simulink model "BMS_V4"  (R2017b)
settings: Solver=FixedStepDiscrete  StartTime=0.0  StopTime=inf  FixedStep=BASETIME  RelTol=1e-3  EnableMultiTasking=on
values from neighbouring files (symbols this model uses):
  AKT_BALANCE = uint16(8)    [BMS_V4_config.m]
  BALANCE = uint16(4)    [BMS_V4_config.m]
  BALANCE_RESISTOR = int32(5)    [BMS_V4_config.m]
  BALANCE_VEC = uint16(8)    [BMS_V4_config.m]
  CELL_SOC = uint16(7)    [BMS_V4_config.m]
  CELL_STATE = uint16(3)    [BMS_V4_config.m]
  CELL_TEMPERATURE = uint16(6)    [BMS_V4_config.m]
  CELL_VOLTAGE = uint16(5)    [BMS_V4_config.m]
  CELLACTBITFIELD = hex2dec('300')    [BMS_V4_config.m]
  CELLDEACTBITFIELD = hex2dec('100')    [BMS_V4_config.m]
  CELLT_BURST = uint16(6)    [BMS_V4_config.m]
  CELLV_BURST = uint16(5)    [BMS_V4_config.m]
  CLK_CYC_timer_1 = 586    [BMS_V4_config.m]
  CLK_CYC_timer_2 = 5860    [BMS_V4_config.m]
  CLK_CYC_timer_3 = 280    [BMS_V4_config.m]
  CLK_CYC_timer_4 = 586*100    (= 58600)    [BMS_V4_config.m]
  CLK_CYC_timer_5 = 5800*2    (= 11600)    [BMS_V4_config.m]
  CLK_CYC_timer_6 = 320    [BMS_V4_config.m]
  CN_CELLS = int32(40*3600)    [BMS_V4_config.m]
  CONTACTOR = uint16(1)    [BMS_V4_config.m]
  CONTACTOR_LOCKED = uint16(0)    [BMS_V4_config.m]
  CONTACTOR_UNLOCKED = uint16(1)    [BMS_V4_config.m]
  DEBUG_SEND_STATES = uint16(hex2dec('01'))    [BMS_V4_config.m]
  DELTA_SOC_BALANCE = int32(5*1e6)    [BMS_V4_config.m]
  DELTA_SOC_BALANCE_OFF = int32(1*1e5)    [BMS_V4_config.m]
  DETERMINE_MODEL_PARAMETER_ACT = uint16(100)    [BMS_V4_config.m]
  DETERMINE_MODEL_PARAMETER_SCC = uint16(101)    [BMS_V4_config.m]
  ERROR = uint16(1)    [BMS_V4_config.m]
  EXTERN_SIGNALS = uint16(1)    [BMS_V4_config.m]
  FREQUENCY_STEPS = uint16([25 50 75 100 150 250 500 750                                      1000 1500 2500 5000 7500                                      10010 10015 10025 10050 10075                                      10100 10150 10250 10500 10750                                      11000 11500])    [BMS_V4_config.m]
  GET_IMAG_PART_MFC = uint16(9)    [BMS_V4_config.m]
  GET_IMAG_PART_MSF = uint16(4)    [BMS_V4_config.m]
  GET_REAL_PART_MFC = uint16(8)    [BMS_V4_config.m]
  GET_REAL_PART_MSF = uint16(3)    [BMS_V4_config.m]
  IMU = uint16(7)    [BMS_V4_config.m]
  IMU_AMP_OFF = uint16(5)    [BMS_V4_config.m]
  IMU_DATA_READ_LOCUS_ACT = uint16(6)    [BMS_V4_config.m]
  IMU_DATA_READ_LOCUS_SCC = uint16(7)    [BMS_V4_config.m]
  IMU_DEBUG = uint16(9)    [BMS_V4_config.m]
  IMU_GET_DATA_MFC = uint16(8)    [BMS_V4_config.m]
  IMU_GET_DATA_MSF = uint16(3)    [BMS_V4_config.m]
  IMU_OFFSET_POLLING = uint16(11)    [BMS_V4_config.m]
  IMU_POLLING = uint16(2)    [BMS_V4_config.m]
  IMU_POWER = uint16(10)    [BMS_V4_config.m]
  IMU_SEND_IMAG = uint16(11)    [BMS_V4_config.m]
  IMU_SEND_REAL = uint16(10)    [BMS_V4_config.m]
  INDEX_IMAGPART = uint16(2)    [BMS_V4_config.m]
  INDEX_REALPART = uint16(1)    [BMS_V4_config.m]
  INFO = uint16(2)    [BMS_V4_config.m]
  INIT_OFFSET_AMPLITUDE = uint16(2)    [BMS_V4_config.m]
  LINE_CURRENT = uint16(3)    [BMS_V4_config.m]
  LINE_CURRENT_CANA = uint16(4)    [BMS_V4_config.m]
  LINE_CURRENT_SWITCH_THRESHOLD = int32(2*1e6)    [BMS_V4_config.m]
  NUM_OF_CELLS = uint16(16)    [BMS_V4_config.m]
  NUM_OF_FREQUENCIES_PSO = uint16(14)    [BMS_V4_config.m]
  NUM_OF_LINES = uint16(1)    [BMS_V4_config.m]
  NUM_OF_PARAMETER = single(5)    [BMS_V4_config.m]
  NUM_OF_SOC_POINTS = uint16(110)    [BMS_V4_config.m]
  P_L_BOUND = single([0.05;0.01;0.1;0.01;0.1])    [BMS_V4_config.m]
  P_U_BOUND = single([0.50;0.20;0.9;0.06;60])    [BMS_V4_config.m]
  PARA_ACT_SEND = uint16(101)    [BMS_V4_config.m]
  PARA_DATA_STORE_ACT = uint16(8)    [BMS_V4_config.m]
  PARA_DATA_STORE_SCC = uint16(9)    [BMS_V4_config.m]
  PARA_SCC_SEND = uint16(102)    [BMS_V4_config.m]
  PARTICLE_INIT = single(create_startparticle(P_L_BOUND,P_U_BOUND,NUM_OF_PARTICLE))    [BMS_V4_config.m]
  POLACT = hex2dec('00000BFF')    [BMS_V4_config.m]
  POLDEACT = hex2dec('000008FF')    [BMS_V4_config.m]
  PSO_PARA_DEBUG = uint16(13)    [BMS_V4_config.m]
  REQUEST_SOC_REF = uint16(1000)    [BMS_V4_config.m]
  SCALE_FACTOR_CH1 = single(0.66666666)    [BMS_V4_config.m]
  SCALE_FACTOR_CH2 = single(0.66666666)    [BMS_V4_config.m]
  SEND_CELL_SOC_ABS = uint16(199)    [BMS_V4_config.m]
  SHUT_DOWN_BALANCE_OFF = uint16(3)    [BMS_V4_config.m]
  SHUT_DOWN_BALANCE_ON = uint16(2)    [BMS_V4_config.m]
  START_IMU_MSL = uint16(3)    [BMS_V4_config.m]
  START_IMU_SCC = uint16(1)    [BMS_V4_config.m]
  SWITCH_IMU_OFF = uint16(2)    [BMS_V4_config.m]
  SWITCH_IMU_ON = uint16(1)    [BMS_V4_config.m]
  SWITCH_IMU_ON_OFF = uint16(4)    [BMS_V4_config.m]
  SYSTEM_DEBUG = uint16(12)    [BMS_V4_config.m]
  TIMEOUT_CANA = uint32(5000)    [BMS_V4_config.m]
  TIMEOUT_GATEWAY = uint32(500)    [BMS_V4_config.m]
  TS_SOC = single(0.010)    [BMS_V4_config.m]
  WARNING = uint16(2)    [BMS_V4_config.m]
libraries: c280xlib x44, c2833xlib x5, simulink x2, c2000lib x1, idelinklib_common x1
(part 4 of 8)

== matlab function BMS_V4/FunctionCall_CANA_send/send_control_CANA ==
  data: error_enable output; CAN_error_low output uint32; CAN_error_high output uint32; warning_enable output; CAN_warning_low output; CAN_warning_high output; cell_states_enable output boolean; CAN_cell_states_low output uint32; CAN_cell_states_high output uint32; line_current_enable output boolean; CAN_line_current_low output uint32; CAN_line_current_high output uint32; cellV_enable output boolean; CAN_cellV_low output uint32; CAN_cellV_high output uint32; cellT_enable output boolean; CAN_cellT_low output uint32; CAN_cellT_high output uint32; cell_SOC_enable output boolean; CAN_cell_SOC_low output uint32; CAN_cell_SOC_high output uint32; balance_enable output boolean; CAN_balance_low output uint32; CAN_balance_high output uint32; timer_ms data_store_memory; NUM_OF_CELLS parameter; NUM_OF_LINES parameter; TIMEOUT_CANA parameter; ERROR parameter; CELL_STATE parameter; LINE_CURRENT_CANA parameter; CELL_VOLTAGE parameter; CELL_TEMPERATURE parameter; CELL_SOC parameter; BALANCE_VEC parameter; CANA_send_data data_store_memory; cell_temperatures data_store_memory; cell_soc_CC data_store_memory; line_currents data_store_memory; IMU_DEBUG parameter; IMU_SEND_REAL parameter; IMU_SEND_IMAG parameter; imu_debug_enable output boolean; CAN_imu_debug_low output uint32; CAN_imu_debug_high output uint32; imu_debug_CAN_low data_store_memory; imu_debug_CAN_high data_store_memory; imu_send_meas_data data_store_memory; imu_state data_store_memory; imu_mfc_state data_store_memory; imu_offset_is_set data_store_memory; imu_on_off data_store_memory; DEBUG_SEND_STATES parameter; imu_in_progress data_store_memory; imu_send_real_enable output boolean; CAN_imu_real_low output uint32; CAN_imu_real_high output uint32; imu_send_imag_enable output boolean; CAN_imu_imag_low output uint32; CAN_imu_imag_high output uint32; system_debug_enable output boolean; CAN_system_debug_low output uint32; CAN_system_debug_high output uint32; ga_parameter_enable output boolean; CAN_ga_parameter_low output uint32; CAN_ga_parameter_high output uint32; parameter_one_cell_scc data_store_memory; PSO_PARA_DEBUG parameter; determined_soc_ga_alpha data_store_memory; determined_soc_ga_rd data_store_memory; cell_voltages data_store_memory; WARNING parameter; error_state data_store_memory; warning_state data_store_memory; cell_states data_store_memory; SYSTEM_DEBUG parameter; REQUEST_SOC_REF parameter; soc_ref_required data_store_memory; soc_ref_in_progress data_store_memory; system_debug_request data_store_memory; balance_vector data_store_memory; para_send_act_cell_CANA data_store_memory; para_send_act_or_scc_CANA data_store_memory; PARA_ACT_SEND parameter; PARA_SCC_SEND parameter; parameter_one_cell_act data_store_memory; NUM_OF_SOC_POINTS parameter; last_soc_point_index data_store_memory; soc_points_of_scc data_store_memory; soc_of_one_para_act data_store_memory; cell_soc_ABS data_store_memory; SEND_CELL_SOC_ABS parameter; active_balance_vector data_store_memory
function [ error_enable, CAN_error_low, CAN_error_high,...
    warning_enable, CAN_warning_low, CAN_warning_high,...
  cell_states_enable, CAN_cell_states_low, CAN_cell_states_high,...
  line_current_enable,CAN_line_current_low, CAN_line_current_high,...
  cellV_enable, CAN_cellV_low, CAN_cellV_high,...
  cellT_enable, CAN_cellT_low, CAN_cellT_high,...
  cell_SOC_enable, CAN_cell_SOC_low, CAN_cell_SOC_high,...
  balance_enable, CAN_balance_low, CAN_balance_high,...
  imu_debug_enable, CAN_imu_debug_low, CAN_imu_debug_high,...
  imu_send_real_enable, CAN_imu_real_low, CAN_imu_real_high,...
  imu_send_imag_enable, CAN_imu_imag_low, CAN_imu_imag_high,...
  system_debug_enable, CAN_system_debug_low, CAN_system_debug_high,...
  ga_parameter_enable, CAN_ga_parameter_low, CAN_ga_parameter_high]...
 = Send_control_CANA...
    (NUM_OF_CELLS, NUM_OF_LINES, TIMEOUT_CANA, ERROR, CELL_STATE,...
    LINE_CURRENT_CANA, CELL_VOLTAGE, CELL_TEMPERATURE,...
    CELL_SOC, BALANCE_VEC,IMU_DEBUG,IMU_SEND_REAL,IMU_SEND_IMAG,...
    DEBUG_SEND_STATES,PSO_PARA_DEBUG, WARNING, SYSTEM_DEBUG,...
    REQUEST_SOC_REF, PARA_ACT_SEND, PARA_SCC_SEND, NUM_OF_SOC_POINTS, SEND_CELL_SOC_ABS)

global CANA_send_data;
global timer_ms;
global cell_voltages;
global cell_temperatures;
global cell_soc_CC;
global line_currents;
global imu_debug_CAN_low;
global imu_debug_CAN_high;
global imu_send_meas_data;
global imu_state;
global imu_mfc_state;
global imu_offset_is_set;
global imu_on_off;
global imu_in_progress;
global parameter_one_cell_scc;
global parameter_one_cell_act;
global determined_soc_ga_alpha;
global determined_soc_ga_rd;
global error_state;
global warning_state;
global cell_states;
global soc_ref_required;
global soc_ref_in_progress;
global system_debug_request;
global balance_vector;
global para_send_act_cell_CANA;
global para_send_act_or_scc_CANA;
global last_soc_point_index;
global soc_points_of_scc;
global soc_of_one_para_act;
global cell_soc_ABS;

global active_balance_vector;

persistent timer_old;
if isempty(timer_old)
    timer_old = uint32(0);
end

persistent cell_no_volt;
if isempty(cell_no_volt)
    cell_no_volt = uint16(1);
end

persistent cell_no_temp;
if isempty(cell_no_temp)
    cell_no_temp = uint16(1);
end

persistent cell_no_soc_cc;
if isempty(cell_no_soc_cc)
    cell_no_soc_cc = uint16(1);
end

persistent cell_no_cell_state;
if isempty(cell_no_cell_state)
    cell_no_cell_state = uint16(1);
end

persistent cell_no_pso;
if isempty(cell_no_pso)
    cell_no_pso = uint16(1);
end

persistent soc_point_scc;
if isempty(soc_point_scc)
    soc_point_scc = uint16(1);
end

persistent para_index;
if isempty(para_index)
    para_index = uint16(1);
end


persistent next_msg;
if isempty(next_msg)
    next_msg = true;
end

 
 persistent e_state;
 if isempty(e_state)
     e_state = uint16([0 0]);
 end
 
 persistent act_balance_count;
 if isempty(act_balance_count)
     act_balance_count = uint32(1);
 end
 

CAN_cellV_high = uint32(0);
CAN_cellV_low = uint32(0);
CAN_cellT_high = uint32(0);
CAN_cellT_low = uint32(0);
CAN_line_current_high = uint32(0);
CAN_line_current_low = uint32(0);
CAN_cell_states_high = uint32(0);
CAN_cell_states_low = uint32(0);
CAN_error_high = uint32(0);
CAN_error_low = uint32(0);
CAN_warning_high = uint32(0);
CAN_warning_low = uint32(0);
CAN_cell_SOC_low = uint32(0);
CAN_cell_SOC_high = uint32(0);
CAN_balance_low = uint32(0);
CAN_balance_high = uint32(0);
CAN_imu_debug_low = uint32(0);
CAN_imu_debug_high = uint32(0);
CAN_imu_real_low = uint32(0);
CAN_imu_real_high = uint32(0);
CAN_imu_imag_low = uint32(0);
CAN_imu_imag_high = uint32(0);
CAN_system_debug_low = uint32(0);
CAN_system_debug_high = uint32(0);
CAN_ga_parameter_low = uint32(0);
CAN_ga_parameter_high = uint32(0);

imu_debug_enable =false;
cell_SOC_enable = false;
balance_enable = false;
cellT_enable = false;
line_current_enable = false;
warning_enable = false;
error_enable = false;
cell_states_enable = false;
cellV_enable = false;
imu_send_real_enable  = false;
imu_send_imag_enable  = false;
system_debug_enable  = false;
ga_parameter_enable  = false;

if(next_msg == true)                                                   
    timer_old = timer_ms;
    %if (CANA_send_data(ERROR) == true)
    if (true)
        if( error_state(1) < uint16(hex2dec('FFFE')))
          e_state(1)=error_state(1);
        end
        if( error_state(2) < uint16(hex2dec('FFFE')))
          e_state(2)=error_state(2);
        end
        % error
        CAN_error_high = uint32(bitshift(uint32(e_state(2)),16));        
        CAN_error_low = uint32(e_state(1));  
        error_enable = true;
    end   
   %if (CANA_send_data(WARNING) == true)
    if (true)
        % warning
        CAN_warning_high = uint32(bitshift(uint32(warning_state(2)),16));
        CAN_warning_low = uint32(warning_state(1));  
        warning_enable = true;
        CANA_send_data(WARNING) = false;
    end  
    % cell_states 
    if (CANA_send_data(CELL_STATE) == true)  
         % cell_states 
         line_no = uint16(1);
         
         CAN_cell_states_high = cell_states(cell_no_cell_state,line_no);
         CAN_cell_states_low = uint32(bitor(uint16(line_no),...
            bitshift(uint16(cell_no_cell_state),8)));
                             
       if (cell_no_cell_state+uint16(1) > NUM_OF_CELLS)
            % all states are send
            CANA_send_data(CELL_STATE) = false;
            cell_no_cell_state = uint16(1);
        else
            % next states for next iteration
            cell_no_cell_state = cell_no_cell_state+uint16(1);
       end
        
        cell_states_enable = true;   
      
    end
    if (CANA_send_data(LINE_CURRENT_CANA) == true)
        % line current
        line_no = uint32(1);
        current = typecast(line_currents(line_no),'uint32');
        CAN_line_current_low = uint32(line_no);
        CAN_line_current_high = uint32(current);
        line_current_enable = true;
        CANA_send_data(LINE_CURRENT_CANA) = false;   
      
    end    
    if (CANA_send_data(CELL_VOLTAGE) == true)
        % cell voltages
        
        line_no = uint16(1);
        x1 = uint16(bitor(uint32(line_no),...
            bitshift(uint32(cell_no_volt),8)));
        x2 = uint32(bitor(uint32(x1),...
            bitshift(uint32(cell_voltages(cell_no_volt,line_no)),16)));
        if(cell_no_volt+uint16(1)> NUM_OF_CELLS)% fertig
            x3 = uint32(0);
        elseif(cell_no_volt+uint16(2)> NUM_OF_CELLS)% fertig
            x3 = uint32(cell_voltages(cell_no_volt+uint16(1),line_no));
        else 
            x3 = uint32(bitor(...
                uint32(cell_voltages(cell_no_volt+uint16(1),line_no)),...
                bitshift(uint32(cell_voltages(cell_no_volt+uint16(2),...
                line_no)),16)));
        end
            
        CAN_cellV_high  = x3;
        CAN_cellV_low   = x2;
        cellV_enable    = true;       
       if (cell_no_volt+uint16(3) > NUM_OF_CELLS)
            % all voltages are send
            CANA_send_data(CELL_VOLTAGE) = false;
            cell_no_volt = uint16(1);
        else
            % next voltage for next iteration
            cell_no_volt=cell_no_volt+uint16(3);
        end

    end    
    if (CANA_send_data(CELL_TEMPERATURE) == true)
        % cell temperatures
        line_no = uint16(1);
        x1 = uint16(bitor(uint16(line_no),...
            bitshift(uint16(cell_no_temp),8)));
        
        temp1=typecast(cell_temperatures(cell_no_temp,line_no),'uint16');
        x2 = uint32(bitor(uint32(x1),...
            bitshift(uint32(temp1),16)));
        
        if(cell_no_temp+uint16(1)> NUM_OF_CELLS)% fertig
            x3 = uint32(0);
        elseif(cell_no_temp+uint16(2)> NUM_OF_CELLS)% fertig
            temp2=typecast(cell_temperatures(cell_no_temp+uint16(1),line_no),'uint16');
            x3 = uint32(temp2);
        else
            temp2=typecast(cell_temperatures(cell_no_temp+uint16(1),line_no),'uint16');
            temp3=typecast(cell_temperatures(cell_no_temp+uint16(2),line_no),'uint16');
            x3 = uint32(bitor(uint32(temp2),bitshift(uint32(temp3),16)));
        end
        CAN_cellT_high = x3;
        CAN_cellT_low  = x2;
        cellT_enable = true;       
       if (cell_no_temp+uint16(3) > NUM_OF_CELLS)
            % all temperatures are send
            CANA_send_data(CELL_TEMPERATURE) = false;
            cell_no_temp = uint16(1);
        else
            % next temperatures for next iteration
            cell_no_temp=cell_no_temp+uint16(3);
       end
    end    
    if (CANA_send_data(CELL_SOC) == true)
        % cell SOC
        % convert from 1Bit = 1u% to 1 Bit = 0.01% 
        line_no = uint16(1);
        
        soc1 = int16(cell_soc_CC(cell_no_soc_cc,line_no)/1e4);
        if(cell_no_soc_cc+uint16(1)> NUM_OF_CELLS)% fertig
            soc2 = int16(0);
            soc3 = int16(0);
        elseif(cell_no_soc_cc+uint16(2)> NUM_OF_CELLS)% fertig
           soc2 = int16(cell_soc_CC(cell_no_soc_cc+uint16(1),line_no)/1e4);
            soc3 = int16(0);
        else
            soc2 = int16(cell_soc_CC(cell_no_soc_cc+uint16(1),line_no)/1e4);
            soc3 = int16(cell_soc_CC(cell_no_soc_cc+uint16(2),line_no)/1e4);
        end
        soc_1_unit = typecast(soc1,'uint16');
        soc_2_unit = typecast(soc2,'uint16');
        soc_3_unit = typecast(soc3,'uint16');
        
        x1 = uint16(bitor(uint16(line_no),...
            bitshift(uint16(cell_no_soc_cc),8)));
        x2 = uint32(bitor(uint32(x1),...
            bitshift(uint32(soc_1_unit),16)));
        x3 = uint32(bitor(uint32(soc_2_unit),...
            bitshift(uint32(soc_3_unit),16)));
        
        CAN_cell_SOC_high   = x3;
        CAN_cell_SOC_low    = x2;
        cell_SOC_enable     = true;       
       if (cell_no_soc_cc+uint16(3) > NUM_OF_CELLS)
            % all soc are send
            CANA_send_data(CELL_SOC) = false;
            cell_no_soc_cc = uint16(1);
        else
            % next soc for next iteration
            cell_no_soc_cc=cell_no_soc_cc+uint16(3);
       end
       
    end    
    if (CANA_send_data(BALANCE_VEC) == true)
        % balance vector
        
       switch act_balance_count
           case 0
                line_nr = uint16(0);
                CAN_balance_low = uint32(line_nr);
                  
                for i = 1:1:NUM_OF_CELLS
                    CAN_balance_low = uint32(bitor(CAN_balance_low,uint32...
                (bitshift(uint32(balance_vector(i)),15+i))));
           
                end
          %      CAN_balance_high_ = uint32(act_balance_count);
                act_balance_count = uint32(1);
                
           case 1       %Output of Cells that need Active Balancing 
               line_nr = uint16(0);
               CAN_balance_low = uint32(line_nr);
               
               for i = 1:1:NUM_OF_CELLS
                    CAN_balance_low = uint32(bitor(CAN_balance_low,uint32...
                    (bitshift(uint32(active_balance_vector(i,act_balance_count)),15+i))));
             
               end 
          %     CAN_balance_high_ = uint32(act_balance_count);
               act_balance_count = uint32(2);
           
               
           case 2       %Output of needed Energy for Active Balancing (just MAX)
               line_nr = uint16(0);
               CAN_balance_low = uint32(line_nr);
               
               
                    CAN_balance_low = uint32(bitor(CAN_balance_low,uint32...
                    (bitshift(uint32(max(active_balance_vector(:,act_balance_count))),16))));
             
                
           %    CAN_balance_high_ = uint32(act_balance_count);
               act_balance_count = uint32(3);
               
           case 3       %Output of Cells with activated Active Balancing
               line_nr = uint16(0);
               CAN_balance_low = uint32(line_nr);
               
               for i = 1:1:NUM_OF_CELLS
                    CAN_balance_low = uint32(bitor(CAN_balance_low,uint32...
                    (bitshift(uint32(active_balance_vector(i,act_balance_count)),15+i))));
             
               end 
           %    CAN_balance_high_ = uint32(act_balance_count);
               act_balance_count = uint32(4);
               
           case 4       %Output of charged Energy for Active Balancing
               line_nr = uint16(0);
               CAN_balance_low = uint32(line_nr);
                             
               CAN_balance_low = uint32(bitor(CAN_balance_low,uint32...
               (bitshift(uint32(max(active_balance_vector(:,act_balance_count))),16))));
             
                
             %  CAN_balance_high_ = uint32(act_balance_count);
               act_balance_count = uint32(0);
               
           otherwise       % Set control variable to init value
                CAN_balance_low = uint32(0);
            %    CAN_balance_high_ = uint32(act_balance_count);
                act_balance_count = uint32(0);
           
           
       end
       
        CAN_balance_high = uint32(act_balance_count);
         balance_enable = true;
         
         
        CANA_send_data(BALANCE_VEC) = false;
    
    end    
    if ((CANA_send_data(IMU_DEBUG) == true) &&...
            (imu_send_meas_data == false))
            CODE = uint16([DEBUG_SEND_STATES 0 0 0 0 0 0 0]);
            CODE(2)= imu_state; 
            CODE(3)= uint16(0);  % to be implemented msf_state; 
            CODE(4)= imu_mfc_state;
            CODE(5)= imu_offset_is_set;
            CODE(6)= imu_on_off;
            CODE(7)= imu_in_progress; 
            CODE(8)= uint16(0);  % to be implemented imu queue;;
            x1=uint16(bitand(uint16(hex2dec('00ff')),uint16(CODE(1))));
            x2=uint16(bitand(uint16(hex2dec('ff00')),uint16(bitshift(uint16(CODE(2)),8))));
            x3=uint16(bitand(uint16(hex2dec('00ff')),uint16(CODE(3))));
            x4=uint16(bitand(uint16(hex2dec('ff00')),uint16(bitshift(uint16(CODE(4)),8))));
            x11=uint16(bitor(x1,x2));
            x12=uint16(bitor(x3,x4));
            CAN_imu_debug_low=uint32(bitor(uint32(x11),bitshift(uint32(x12),16)));
            
            x5=uint16(bitand(uint16(hex2dec('00ff')),uint16(CODE(5))));
            x6=uint16(bitand(uint16(hex2dec('ff00')),uint16(bitshift(uint16(CODE(6)),8))));
            x7=uint16(bitand(uint16(hex2dec('00ff')),uint16(CODE(7))));
            x8=uint16(bitand(uint16(hex2dec('ff00')),uint16(bitshift(uint16(CODE(8)),8))));
            x21=uint16(bitor(x5,x6));
            x22=uint16(bitor(x7,x8));
            
            CAN_imu_debug_high=uint32(bitor(uint32(x21),bitshift(uint32(x22),16)));
        
         imu_debug_enable = true;
        CANA_send_data(IMU_DEBUG) = false;  
        
    end    
    if (CANA_send_data(IMU_SEND_REAL) == true)
         CAN_imu_real_low  = imu_debug_CAN_low;
         CAN_imu_real_high = imu_debug_CAN_high;
       
         imu_send_real_enable = true;
         CANA_send_data(IMU_SEND_REAL) = false;
     
    end    
    if (CANA_send_data(IMU_SEND_IMAG) == true)
         CAN_imu_imag_low  = imu_debug_CAN_low;
         CAN_imu_imag_high = imu_debug_CAN_high;
       
         imu_send_imag_enable = true;
         CANA_send_data(IMU_SEND_IMAG) = false;
         
    end  
    if (CANA_send_data(SYSTEM_DEBUG) == true)
            
         switch system_debug_request
             case REQUEST_SOC_REF
                 x1=uint16(bitand(uint16(hex2dec('00ff')),...
                     uint16(soc_ref_required)));
                 x2=uint16(bitand(uint16(hex2dec('ff00')),...
                     uint16(bitshift(uint16(soc_ref_in_progress),8))));
                 x11 =uint16(bitor(x1,x2));
                 CAN_system_debug_low =...
                     uint32(bitor(uint32(REQUEST_SOC_REF),...
                     bitshift(uint32(x11),16)));
                 CAN_system_debug_high = uint32(0);
             case SEND_CELL_SOC_ABS
                 soc_abs = int16(cell_soc_ABS/1e5); % 0.0%->6500.3%
                 soc_abs_uint = typecast(soc_abs,'uint16');
                 
                 CAN_system_debug_low = uint32(SEND_CELL_SOC_ABS);
                 CAN_system_debug_high = uint32(soc_abs_uint);
                 
         end
         system_debug_enable = true;
         CANA_send_data(SYSTEM_DEBUG) = false;
    end
    if (CANA_send_data(PSO_PARA_DEBUG) == true)
        % model parameter
        %line_no = uint16(1);
        ga_parameter_enable  = true;  
        switch para_send_act_or_scc_CANA
            case PARA_SCC_SEND
                cell_no_pso = para_send_act_cell_CANA;
                switch para_index
                    case 1%RS
                        value_s = parameter_one_cell_scc(soc_point_scc,1);
                        x1=uint32(bitand(uint32(hex2dec('000000ff')),...
                            uint32(11)));
                        x2=uint32(bitand(uint32(hex2dec('0000ff00')),...
                            uint32(bitshift(uint32(cell_no_pso),8))));
                        x3=uint32(bitand(uint32(hex2dec('00ff0000')),...
                            uint32(bitshift(uint32(soc_point_scc),16))));
                        x11 = uint32(bitor(x1,x2));
                        CAN_ga_parameter_low = uint32(bitor(x11,x3));
                        CAN_ga_parameter_high = typecast(value_s,'uint32'); 
                    case 2 %RD
                        value_s = parameter_one_cell_scc(soc_point_scc,2);
                        x1=uint32(bitand(uint32(hex2dec('000000ff')),...
                            uint32(12)));
                        x2=uint32(bitand(uint32(hex2dec('0000ff00')),...
                            uint32(bitshift(uint32(cell_no_pso),8))));
                        x3=uint32(bitand(uint32(hex2dec('00ff0000')),...
                            uint32(bitshift(uint32(soc_point_scc),16))));
                        x11 = uint32(bitor(x1,x2));
                        CAN_ga_parameter_low = uint32(bitor(x11,x3));
                        CAN_ga_parameter_high = typecast(value_s,'uint32'); 
                    case 3 %alpha
                        value_s = parameter_one_cell_scc(soc_point_scc,3);
                        x1=uint32(bitand(uint32(hex2dec('000000ff')),...
                            uint32(13)));
                        x2=uint32(bitand(uint32(hex2dec('0000ff00')),...
                            uint32(bitshift(uint32(cell_no_pso),8))));
                        x3=uint32(bitand(uint32(hex2dec('00ff0000')),...
                            uint32(bitshift(uint32(soc_point_scc),16))));
                        x11 = uint32(bitor(x1,x2));
                        CAN_ga_parameter_low = uint32(bitor(x11,x3));
                        CAN_ga_parameter_high = typecast(value_s,'uint32'); 
                    case 4 %k
                        value_s = parameter_one_cell_scc(soc_point_scc,4);
                        x1=uint32(bitand(uint32(hex2dec('000000ff')),...
                            uint32(14)));
                        x2=uint32(bitand(uint32(hex2dec('0000ff00')),...
                            uint32(bitshift(uint32(cell_no_pso),8))));
                        x3=uint32(bitand(uint32(hex2dec('00ff0000')),...
                            uint32(bitshift(uint32(soc_point_scc),16))));
                        x11 = uint32(bitor(x1,x2));
                        CAN_ga_parameter_low = uint32(bitor(x11,x3));
                        CAN_ga_parameter_high = typecast(value_s,'uint32'); 
                    case 5 %wg
                        value_s = parameter_one_cell_scc(soc_point_scc,5);
                        x1=uint32(bitand(uint32(hex2dec('000000ff')),...
                            uint32(15)));
                        x2=uint32(bitand(uint32(hex2dec('0000ff00')),...
                            uint32(bitshift(uint32(cell_no_pso),8))));
                        x3=uint32(bitand(uint32(hex2dec('00ff0000')),...
                            uint32(bitshift(uint32(soc_point_scc),16))));
                        x11 = uint32(bitor(x1,x2));
                        CAN_ga_parameter_low = uint32(bitor(x11,x3));
                        CAN_ga_parameter_high = typecast(value_s,'uint32'); 
                    case 6 %L2
                        value_s = parameter_one_cell_scc(soc_point_scc,6);
                        x1=uint32(bitand(uint32(hex2dec('000000ff')),...
                            uint32(16)));
                        x2=uint32(bitand(uint32(hex2dec('0000ff00')),...
                            uint32(bitshift(uint32(cell_no_pso),8))));
                        x3=uint32(bitand(uint32(hex2dec('00ff0000')),...
                            uint32(bitshift(uint32(soc_point_scc),16))));
                        x11 = uint32(bitor(x1,x2));
                        CAN_ga_parameter_low = uint32(bitor(x11,x3));
                        CAN_ga_parameter_high = typecast(value_s,'uint32'); 
                     case 7 %SoC value of SCC 
                        value_soc = soc_points_of_scc(soc_point_scc);
                        x1=uint32(bitand(uint32(hex2dec('000000ff')),...
                            uint32(17)));
                        x2=uint32(bitand(uint32(hex2dec('0000ff00')),...
                            uint32(bitshift(uint32(cell_no_pso),8))));
                        x3=uint32(bitand(uint32(hex2dec('00ff0000')),...
                            uint32(bitshift(uint32(soc_point_scc),16))));
                        x11 = uint32(bitor(x1,x2));
                        CAN_ga_parameter_low = uint32(bitor(x11,x3));
                        CAN_ga_parameter_high = typecast(value_soc,'uint32');
%                         value = determined_soc_ga_alpha(cell_no_ga);
%                         CAN_ga_parameter_low  = uint32(bitor(uint16(17),...
%                             bitshift(uint16(cell_no_ga),8))); 
%                         CAN_ga_parameter_high = typecast(value,'uint32');                
%                     case 8
%                         value = determined_soc_ga_rd(cell_no_ga);
%                         CAN_ga_parameter_low  = uint32(bitor(uint16(18),...
%                             bitshift(uint16(cell_no_ga),8))); 
%                         CAN_ga_parameter_high = typecast(value,'uint32');
                end            
                if(para_index >= 7)
                    %if (soc_point_scc >= NUM_OF_SOC_POINTS)
                    if (soc_point_scc >= last_soc_point_index)    
                    % all para are send
                        CANA_send_data(PSO_PARA_DEBUG) = false;
                        soc_point_scc = uint16(1);
                    else
                        soc_point_scc = soc_point_scc+uint16(1);
                    end
                    para_index = uint16(1);
                else
                    para_index = para_index + uint16(1);
                end
                
            case PARA_ACT_SEND
                cell_no_pso = para_send_act_cell_CANA;
                switch para_index
                    case 1%RS
                        value_s = parameter_one_cell_act(1);
                        CAN_ga_parameter_low  = uint32(bitor(uint16(21),...
                            bitshift(uint16(cell_no_pso),8))); 
                        CAN_ga_parameter_high = typecast(value_s,'uint32'); 
                    case 2 %RD
                        value_s = parameter_one_cell_act(2);
                        CAN_ga_parameter_low  = uint32(bitor(uint16(22),...
                            bitshift(uint16(cell_no_pso),8))); 
                        CAN_ga_parameter_high = typecast(value_s,'uint32');
                    case 3 %alpha
                        value_s = parameter_one_cell_act(3);
                        CAN_ga_parameter_low  = uint32(bitor(uint16(23),...
                            bitshift(uint16(cell_no_pso),8))); 
                        CAN_ga_parameter_high = typecast(value_s,'uint32');
                    case 4 %k
                        value_s = parameter_one_cell_act(4);
                        CAN_ga_parameter_low  = uint32(bitor(uint16(24),...
                            bitshift(uint16(cell_no_pso),8))); 
                        CAN_ga_parameter_high = typecast(value_s,'uint32');
                    case 5 %wg
                        value_s = parameter_one_cell_act(5);
                        CAN_ga_parameter_low  = uint32(bitor(uint16(25),...
                            bitshift(uint16(cell_no_pso),8))); 
                        CAN_ga_parameter_high = typecast(value_s,'uint32');
                    case 6 %L2
                        value_s = parameter_one_cell_act(6);
                        CAN_ga_parameter_low  = uint32(bitor(uint16(26),...
                            bitshift(uint16(cell_no_pso),8))); 
                        CAN_ga_parameter_high = typecast(value_s,'uint32');
                    case 7 % SoC value CC at imu meas
                        value_soc = soc_of_one_para_act;
                        CAN_ga_parameter_low  = uint32(bitor(uint16(27),...
                            bitshift(uint16(cell_no_pso),8))); 
                        CAN_ga_parameter_high = typecast(value_soc,'uint32');
%                         value = determined_soc_ga_alpha(cell_no_ga);
%                         CAN_ga_parameter_low  = uint32(bitor(uint16(17),...
%                             bitshift(uint16(cell_no_ga),8))); 
%                         CAN_ga_parameter_high = typecast(value,'uint32');                
%                     case 8
%                         value = determined_soc_ga_rd(cell_no_ga);
%                         CAN_ga_parameter_low  = uint32(bitor(uint16(18),...
%                             bitshift(uint16(cell_no_ga),8))); 
%                         CAN_ga_parameter_high = typecast(value,'uint32');
                end            
                if(para_index >= 7)
                    CANA_send_data(PSO_PARA_DEBUG) = false;
                    para_index = uint16(1);
                    cell_no_pso = uint16(1);
                else
                    para_index = para_index + uint16(1);
                end
        end         
    
    %end
    end
    
else
    
    if((timer_ms-timer_old) > TIMEOUT_CANA)
       next_msg = true; 
        timer_old = timer_ms-uint32(1);
    end
end
